simulink model "clik_inverse"  (R2022b)
settings: Solver=ode1  StartTime=0.0  StopTime=4  FixedStep=0.001  RelTol=1e-3
undefined symbols (not defined in the file or in its folder): DiscIntNeverNeededParam, q0, Tc
settings Model: Creator=Xp  LastModifiedBy=TAARUN
settings SolverCC: AlgebraicLoopSolver=TrustRegion
settings DataIOCC: LimitDataPoints=on  SaveFormat=Array  SignalLoggingSaveFormat=ModelDataLogs  ReturnWorkspaceOutputs=off
settings OptimizationCC: ExpressionDepthLimit=2147483647  InitFltsAndDblsToZero=on  LifeSpan=inf
settings DebuggingCC: SaveWithParameterizedLinksMsg=none  UnderspecifiedInitializationDetection=Classic  MergeDetectMultiDrivingBlocksExec=none  SolverPrmCheckMsg=warning  MultiTaskDSMMsg=warning  MultiTaskCondExecSysMsg=none  FcnCallInpInsideContextMsg=warning  UnconnectedInputMsg=warning  UnconnectedOutputMsg=warning  UnconnectedLineMsg=warning  StateNameClashWarn=warning  SFUnexpectedBacktrackingDiag=warning  SFNoUnconditionalDefaultTransitionDiag=warning  SFExecutionAtInitializationDiag=none  SFMachineParentedDataDiag=warning  ArithmeticOperatorsInVariantConditions=warning
settings HardwareCC: ProdBitPerPointer=32  ProdBitPerSizeT=32  ProdBitPerPtrDiffT=32  ProdLargestAtomicFloat=None  ProdIntDivRoundTo=Undefined  ProdEndianess=Unspecified  ProdWordSize=32  ProdHWDeviceType=32-bit Generic
settings ModelReferenceCC: EnableRefExpFcnMdlSchedulingChecks=on  PropagateSignalLabelsOutOfModel=off
settings SFSimCC: CustomCodeUndefinedFunction=UseInterfaceOnly
settings RTWCC: DLArmComputeVersion=19.05
settings CodeAppCC: StateflowObjectComments=on
settings GRTTargetCC: TargetLangStandard=C89/C90 (ANSI)  CombineOutputUpdateFcns=off  GRTInterface=on
settings ConfigComp: CovMetricSettings=dw  CovSaveCumulativeToWorkspaceVar=on  CovSaveSingleToWorkspaceVar=on

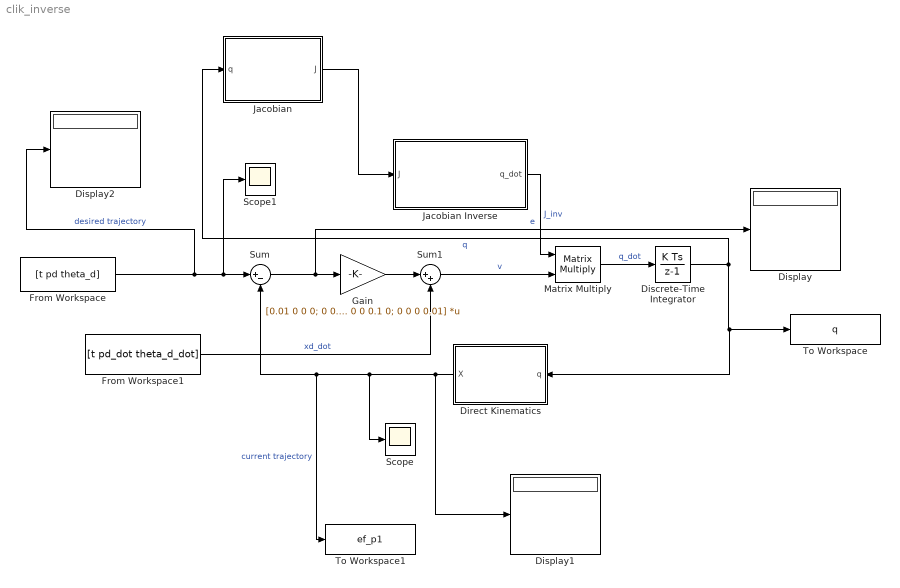
== system clik_inverse ==
  Direct Kinematics : MATLAB Function  TreatAsAtomicUnit=on
  Discrete-Time Integrator : DiscreteIntegrator  InitialCondition=q0  SampleTime=Tc  LimitOutput=on  UpperSaturationLimit=[pi/2; pi/4; 1; 2*pi]  LowerSaturationLimit=[-pi/2; -pi/2; 0.25; -2*pi]  ICPrevOutput=DiscIntNeverNeededParam  ICPrevScaledInput=DiscIntNeverNeededParam
  Display : Display
  Display1 : Display
  Display2 : Display
  From Workspace : FromWorkspace  VariableName=[t pd theta_d]  SampleTime=Tc
  From Workspace1 : FromWorkspace  VariableName=[t pd_dot theta_d_dot]  SampleTime=Tc
  Gain : Gain  Gain=[0.01 0 0 0; 0 0.01 0 0; 0 0 0.1 0; 0 0 0 0.01]  Multiplication=Matrix(K*u)
  Jacobian : MATLAB Function  TreatAsAtomicUnit=on
  Jacobian Inverse : MATLAB Function  TreatAsAtomicUnit=on
  Matrix Multiply : Product  Multiplication=Matrix(*)
  Scope : Scope
  Scope1 : Scope
  Sum : Sum  Inputs=|+-
  Sum1 : Sum  Inputs=|++
  To Workspace : ToWorkspace  VariableName=q  SampleTime=Tc
  To Workspace1 : ToWorkspace  VariableName=ef_p1  SampleTime=Tc
  wires:
  From Workspace/1 -> Display2/1, Scope1/1, Sum/1  "desired trajectory"
  Sum/1 -> Display/1, Gain/1  "e"
  Gain/1 -> Sum1/1
  From Workspace1/1 -> Sum1/2  "xd_dot"
  Discrete-Time Integrator/1 -> To Workspace/1, Direct Kinematics/1(q), Jacobian/1(q)  "q"
  Sum1/1 -> Matrix Multiply/2  "v"
  Matrix Multiply/1 -> Discrete-Time Integrator/1  "q_dot"
  Jacobian Inverse/1(q_dot) -> Matrix Multiply/1  "J_inv"
  Direct Kinematics/1(X) -> Display1/1, Scope/1, To Workspace1/1, Sum/2  "current trajectory"
  Jacobian/1(J) -> Jacobian Inverse/1(J)

== matlab function clik_inverse/Jacobian Inverse ==
  data: J input; q_dot output
function q_dot = compute_jacobian_inverse(J)

q_dot = jacobian_inverse(J);

== matlab function clik_inverse/Direct Kinematics ==
  data: q input; X output
function X = direct_kinematics(q)

X = direct_kin(q);

== matlab function clik_inverse/Jacobian ==
  data: q input; J output
function J = compute_jacobian(q)
    
J = jacobian(q);
